simulink model "dvbs2hdlTransmitter"  (R2024b)
settings: Solver=FixedStepDiscrete  StartTime=0.0  StopTime=stopTime  RelTol=1e-3
InitFcn:
  | dvbs2hdlTxInit;
  | 
  | clear simDummyFrameNos;
StopFcn:
  | if exist('simDummyFrameNos','var')
  |    dvbs2hdlTransmitterVerify;
  | end
undefined symbols (not defined in the file or in its folder): DFLNormal, DFLShort, MODCOD, nFrames, UPL
libraries: hdlsllib x9, simulink x7, dspsrcs4 x6
CloseFcn:
  | clear curFrameBits curnPkts DFL FECFrame frameBits ...
  |     frameEndIn frameNo frameStartIn MODCOD nFrames ...
  |     pktBitsIn pktEndIn pktsSent pktStartIn pktValidIn ...
  |     PLFL Rsym stopTime StreamFormat syncWord TSorGS ...
  |     UPL
  | clear err FECFrameStr ii matframeLen matTxWaveform ...
  |     MSERe MSEIm relativeMSE RRCgain s2Config simDummyFrameNos ...
  |     simDummyFrameNums simTxWaveform tout logsout ...
  |     txObj bitsPerFrame
  | close(figure(1));
  | clear bitsIn DFLNormal DFLShort
settings Model: DataTypeOverride=Off  SimulationMode=accelerator  Creator=The MathWorks, Inc.  LastModifiedBy=daniel
settings SolverCC: AutoInsertRateTranBlk=on  MaxZcPerStep=1
settings DataIOCC: ReturnWorkspaceOutputs=off
settings OptimizationCC: BlockReduction=off  ConditionallyExecuteInputs=off  DefaultParameterBehavior=Inlined  InheritOutputTypeSmallerThanSingle=on  ReuseModelBlockBuffer=off
settings DebuggingCC: AlgebraicLoopMsg=error  SingleTaskRateTransMsg=error  SubsystemReferenceDiagnosticForUnitTest=warning
settings HardwareCC: ProdBitPerPointer=32  ProdBitPerSizeT=32  ProdBitPerPtrDiffT=32  ProdLargestAtomicFloat=None  ProdIntDivRoundTo=Undefined  ProdEndianess=Unspecified  ProdWordSize=32  ProdHWDeviceType=ASIC/FPGA->ASIC/FPGA  TargetBitPerLong=64  TargetBitPerPointer=64  TargetBitPerSizeT=64  TargetBitPerPtrDiffT=64  TargetLongLongMode=on  TargetIntDivRoundTo=Zero  TargetEndianess=LittleEndian  TargetWordSize=64  TargetHWDeviceType=Custom Processor->MATLAB Host Computer  ProdEqTarget=off
settings ModelReferenceCC: EnableRefExpFcnMdlSchedulingChecks=on
settings RTWCC: GPUComputeCapability=3.5  DLArmComputeVersion=19.05

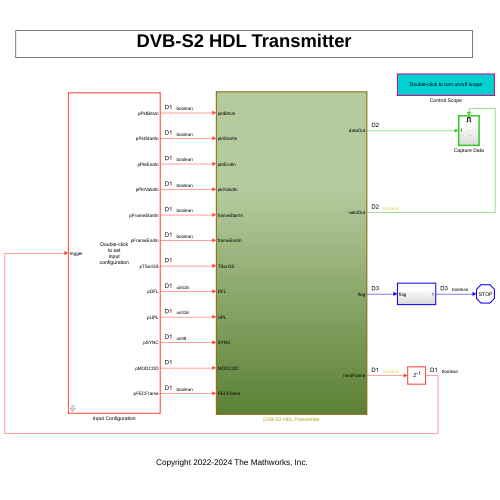
[thumbnail: Simulink's stored preview of the top-level diagram]
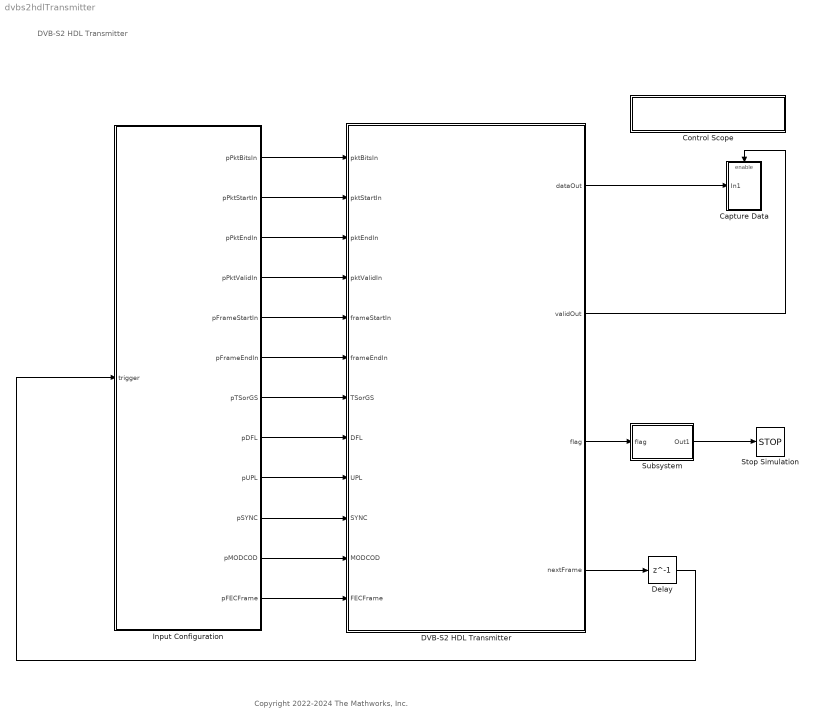
== system dvbs2hdlTransmitter ==
  note: Copyright 2022-2024 The Mathworks, Inc.
  note: DVB-S2 HDL Transmitter
  Capture Data : Subsystem
  Control Scope : Subsystem
      settings: OpenFcn=|
      | h = get_param([gcs '/Capture Data/Spectrum Analyzer'],'ScopeConfiguration');
      | 
      | h.Visible = ~h.Visible;
      | 
      | clear h;
      mask Display: disp('Double-click to turn on/off scope');
  DVB-S2 HDL Transmitter : Subsystem
  Delay : Delay  DelayLength=1
  Input Configuration : Subsystem  mask{Rsym=125e3, MODCODval=[11,17,23,28], FECFrameval=zeros(1,4), InputStreamFormat=GS, UPLval=1504}
      mask prompts: Rsym "Symbol rate:"; MODCODval "MODCOD:"; FECFrameval "FECFrame:"; InputStreamFormat "Input stream format:"; UPLval "UPL:"
      mask TypeOptions InputStreamFormat: TS | GS
      mask DialogControl DescTextVar Prompt: When Input stream format is set to TS, the UPL value is taken as 1504. The value that is set here is ignored.
      mask Display: disp(['Double-click' newline 'to set' newline 'input' newline 'configuration']);
  Stop Simulation : Stop
  Subsystem : Subsystem
      settings: LibrarySourceBlock=|
      | hdlsllib/Ports &
      | Subsystems/Subsystem
  wires:
  Input Configuration/1(pPktBitsIn) -> DVB-S2 HDL Transmitter/1(pktBitsIn)
  Input Configuration/2(pPktStartIn) -> DVB-S2 HDL Transmitter/2(pktStartIn)
  Input Configuration/3(pPktEndIn) -> DVB-S2 HDL Transmitter/3(pktEndIn)
  Input Configuration/4(pPktValidIn) -> DVB-S2 HDL Transmitter/4(pktValidIn)
  Input Configuration/5(pFrameStartIn) -> DVB-S2 HDL Transmitter/5(frameStartIn)
  Input Configuration/6(pFrameEndIn) -> DVB-S2 HDL Transmitter/6(frameEndIn)
  Input Configuration/7(pTSorGS) -> DVB-S2 HDL Transmitter/7(TSorGS)
  Input Configuration/8(pDFL) -> DVB-S2 HDL Transmitter/8(DFL)
  Input Configuration/9(pUPL) -> DVB-S2 HDL Transmitter/9(UPL)
  Input Configuration/10(pSYNC) -> DVB-S2 HDL Transmitter/10(SYNC)
  Input Configuration/11(pMODCOD) -> DVB-S2 HDL Transmitter/11(MODCOD)
  DVB-S2 HDL Transmitter/1(dataOut) -> Capture Data/1(In1)
  DVB-S2 HDL Transmitter/2(validOut) -> Capture Data/Enable
  DVB-S2 HDL Transmitter/4(nextFrame) -> Delay/1
  Input Configuration/12(pFECFrame) -> DVB-S2 HDL Transmitter/12(FECFrame)
  Delay/1 -> Input Configuration/1(trigger)
  DVB-S2 HDL Transmitter/3(flag) -> Subsystem/1(flag)
  Subsystem/1(Out1) -> Stop Simulation/1

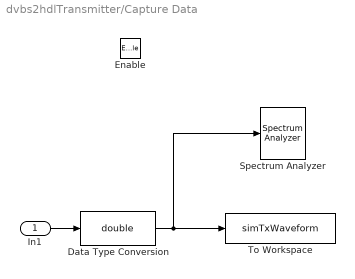
== system dvbs2hdlTransmitter/Capture Data ==
  In1 : Inport
  Enable : EnablePort
  Data Type Conversion : DataTypeConversion  OutDataTypeStr=double  SaturateOnIntegerOverflow=off  RndMeth=Floor
  Spectrum Analyzer : SpectrumAnalyzer  WindowPosition=[267.000000,736.000000,800.000000,450.000000,]  ScopeFrameLocation=window  Span=25000000  StartFrequency=-12500000  StopFrequency=12500000  AveragingMethod=Exponential  YLimits=[-78.80944125,11.88041305]  AllowFFTLengthLessThanSamplesPerUpdate=on
  To Workspace : ToWorkspace  VariableName=simTxWaveform  SampleTime=-1
      settings: Save2DSignal=2-D array (concatenate along first dimension)
  wires:
  In1/1 -> Data Type Conversion/1
  Data Type Conversion/1 -> Spectrum Analyzer/1, To Workspace/1

== system dvbs2hdlTransmitter/Control Scope ==

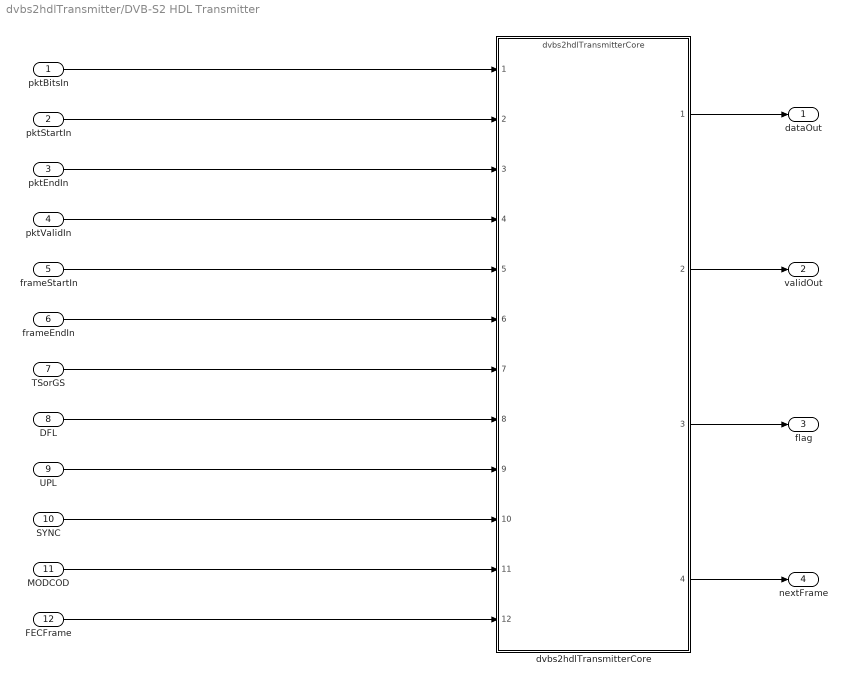
== system dvbs2hdlTransmitter/DVB-S2 HDL Transmitter ==
  pktBitsIn : Inport
  pktStartIn : Inport  Port=2
  pktEndIn : Inport  Port=3
  pktValidIn : Inport  Port=4
  frameStartIn : Inport  Port=5
  frameEndIn : Inport  Port=6
  TSorGS : Inport  Port=7
  DFL : Inport  Port=8
  UPL : Inport  Port=9
  SYNC : Inport  Port=10
  MODCOD : Inport  Port=11
  FECFrame : Inport  Port=12
  dvbs2hdlTransmitterCore : ModelReference  ModelNameDialog=dvbs2hdlTransmitterCore.slx  ModelReferenceVersion=6.8
  dataOut : Outport
  validOut : Outport  Port=2
  flag : Outport  Port=3
  nextFrame : Outport  Port=4
  wires:
  pktBitsIn/1 -> dvbs2hdlTransmitterCore/1
  pktStartIn/1 -> dvbs2hdlTransmitterCore/2
  pktEndIn/1 -> dvbs2hdlTransmitterCore/3
  pktValidIn/1 -> dvbs2hdlTransmitterCore/4
  frameStartIn/1 -> dvbs2hdlTransmitterCore/5
  frameEndIn/1 -> dvbs2hdlTransmitterCore/6
  TSorGS/1 -> dvbs2hdlTransmitterCore/7
  DFL/1 -> dvbs2hdlTransmitterCore/8
  UPL/1 -> dvbs2hdlTransmitterCore/9
  SYNC/1 -> dvbs2hdlTransmitterCore/10
  MODCOD/1 -> dvbs2hdlTransmitterCore/11
  FECFrame/1 -> dvbs2hdlTransmitterCore/12
  dvbs2hdlTransmitterCore/2 -> validOut/1
  dvbs2hdlTransmitterCore/1 -> dataOut/1
  dvbs2hdlTransmitterCore/4 -> nextFrame/1
  dvbs2hdlTransmitterCore/3 -> flag/1

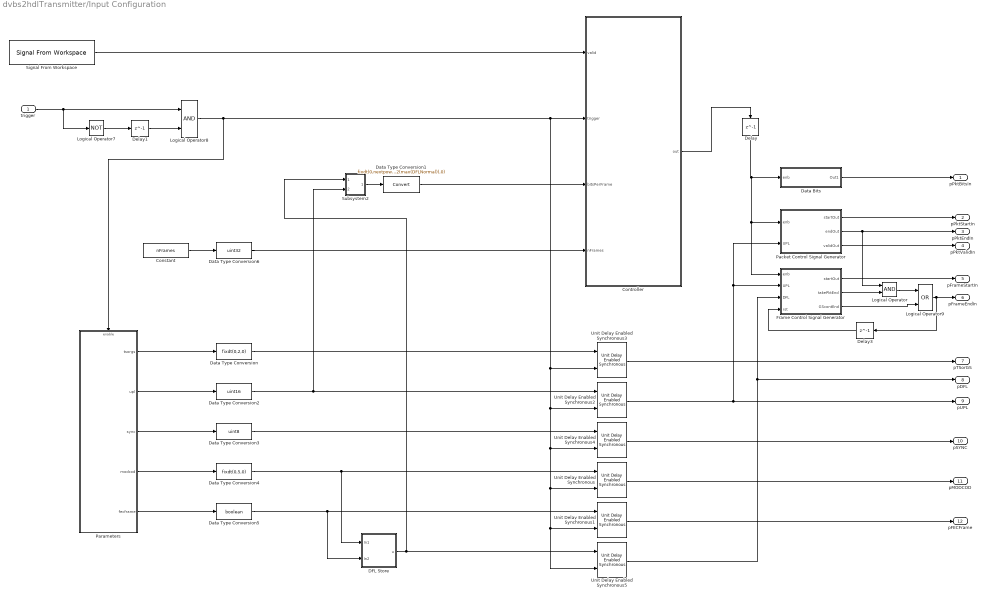
== system dvbs2hdlTransmitter/Input Configuration ==
  trigger : Inport
  Constant : Constant  Value=nFrames  SampleTime=-1
  Controller : MATLAB Function  TreatAsAtomicUnit=on
  DFL Store : Subsystem
  Data Bits : Subsystem
  Data Type Conversion : DataTypeConversion  OutDataTypeStr=fixdt(0,2,0)  SaturateOnIntegerOverflow=off  RndMeth=Floor
  Data Type Conversion1 : DataTypeConversion  OutDataTypeStr=fixdt(0,nextpow2(max(DFLNormal)),0)  SaturateOnIntegerOverflow=off  RndMeth=Floor
  Data Type Conversion2 : DataTypeConversion  OutDataTypeStr=uint16  SaturateOnIntegerOverflow=off  RndMeth=Floor
  Data Type Conversion3 : DataTypeConversion  OutDataTypeStr=uint8  SaturateOnIntegerOverflow=off  RndMeth=Floor
  Data Type Conversion4 : DataTypeConversion  OutDataTypeStr=fixdt(0,5,0)  SaturateOnIntegerOverflow=off  RndMeth=Floor
  Data Type Conversion5 : DataTypeConversion  OutDataTypeStr=boolean  SaturateOnIntegerOverflow=off  RndMeth=Floor
  Data Type Conversion6 : DataTypeConversion  OutDataTypeStr=uint32  SaturateOnIntegerOverflow=off  RndMeth=Floor
  Delay : Delay  DelayLength=1
  Delay1 : Delay  DelayLength=1
  Delay3 : Delay  DelayLength=1
  Frame Control Signal Generator : Subsystem
  Logical Operator : Logic  AllPortsSameDT=off  OutDataTypeStr=boolean
  Logical Operator7 : Logic  Operator=NOT  AllPortsSameDT=off  OutDataTypeStr=boolean
  Logical Operator8 : Logic  AllPortsSameDT=off  OutDataTypeStr=boolean
  Logical Operator9 : Logic  Operator=OR  AllPortsSameDT=off  OutDataTypeStr=boolean
  Packet Control Signal Generator : Subsystem
  Parameters : Subsystem
  Signal From Workspace : dspsrcs4/Signal From Workspace  X=true  Ts=1/(Rsym*8)  nsamps=1  OutputAfterFinalValue=Cyclic repetition  ignoreOrWarnInputAndFrameLengths=off  OutputFrames=off
  Subsystem2 : Subsystem
  Unit Delay Enabled Synchronous{,1..5} (6 alike) : hdlsllib/Discrete/Unit Delay Enabled Synchronous  InitialCondition=0.0  SampleTime=-1
  pPktBitsIn : Outport
  pPktStartIn : Outport  Port=2
  pPktEndIn : Outport  Port=3
  pPktValidIn : Outport  Port=4
  pFrameStartIn : Outport  Port=5
  pFrameEndIn : Outport  Port=6
  pTSorGS : Outport  Port=7
  pDFL : Outport  Port=8
  pUPL : Outport  Port=9
  pSYNC : Outport  Port=10
  pMODCOD : Outport  Port=11
  pFECFrame : Outport  Port=12
  wires:
  Controller/1(out) -> Delay/1
  Data Type Conversion4/1 -> DFL Store/1(In1), Unit Delay Enabled Synchronous/1
  Data Type Conversion5/1 -> Unit Delay Enabled Synchronous1/1, DFL Store/2(In2)
  Data Type Conversion2/1 -> Unit Delay Enabled Synchronous2/1, Subsystem2/2(UPL)
  Signal From Workspace/1 -> Controller/1(valid)
  Unit Delay Enabled Synchronous2/1 -> pUPL/1, Packet Control Signal Generator/2(UPL), Frame Control Signal Generator/2(UPL)
  Frame Control Signal Generator/2(takePktEnd) -> Logical Operator/2
  Packet Control Signal Generator/2(endOut) -> pPktEndIn/1, Logical Operator/1
  Data Type Conversion/1 -> Unit Delay Enabled Synchronous3/1
  Logical Operator8/1 -> Parameters/Enable, Unit Delay Enabled Synchronous3/2, Unit Delay Enabled Synchronous1/2, Unit Delay Enabled Synchronous5/2, Unit Delay Enabled Synchronous/2, Unit Delay Enabled Synchronous4/2, Unit Delay Enabled Synchronous2/2, Controller/2(trigger)
  Data Bits/1(Out1) -> pPktBitsIn/1
  Packet Control Signal Generator/1(startOut) -> pPktStartIn/1
  Packet Control Signal Generator/3(validOut) -> pPktValidIn/1
  Frame Control Signal Generator/1(startOut) -> pFrameStartIn/1
  Logical Operator9/1 -> pFrameEndIn/1, Delay3/1
  Data Type Conversion3/1 -> Unit Delay Enabled Synchronous4/1
  Parameters/2(upl) -> Data Type Conversion2/1
  Parameters/4(modcod) -> Data Type Conversion4/1
  Parameters/5(fecframe) -> Data Type Conversion5/1
  Parameters/1(tsorgs) -> Data Type Conversion/1
  Parameters/3(sync) -> Data Type Conversion3/1
  DFL Store/1(u) -> Subsystem2/1(DFL), Unit Delay Enabled Synchronous5/1
  Unit Delay Enabled Synchronous5/1 -> pDFL/1, Frame Control Signal Generator/3(DFL)
  Unit Delay Enabled Synchronous3/1 -> pTSorGS/1
  Unit Delay Enabled Synchronous/1 -> pMODCOD/1
  Unit Delay Enabled Synchronous4/1 -> pSYNC/1
  Unit Delay Enabled Synchronous1/1 -> pFECFrame/1
  Delay/1 -> Frame Control Signal Generator/1(enb), Packet Control Signal Generator/1(enb), Data Bits/1(enb)
  trigger/1 -> Logical Operator7/1, Logical Operator8/1
  Delay1/1 -> Logical Operator8/2
  Logical Operator7/1 -> Delay1/1
  Delay3/1 -> Frame Control Signal Generator/4(rst)
  Logical Operator/1 -> Logical Operator9/1
  Frame Control Signal Generator/3(GScontEnd) -> Logical Operator9/2
  Constant/1 -> Data Type Conversion6/1
  Data Type Conversion1/1 -> Controller/3(bitsPerFrame)
  Subsystem2/1(Out1) -> Data Type Conversion1/1
  Data Type Conversion6/1 -> Controller/4(nFrames)

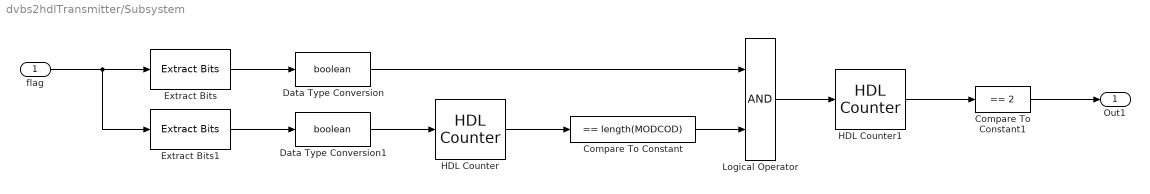
== system dvbs2hdlTransmitter/Subsystem ==
  flag : Inport
  Compare To Constant : simulink/Logic and Bit Operations/Compare To Constant  relop===  const=length(MODCOD)  OutDataTypeStr=boolean
  Compare To Constant1 : simulink/Logic and Bit Operations/Compare To Constant  relop===  const=2  OutDataTypeStr=boolean
  Data Type Conversion : DataTypeConversion  OutDataTypeStr=boolean  SaturateOnIntegerOverflow=off  RndMeth=Floor
  Data Type Conversion1 : DataTypeConversion  OutDataTypeStr=boolean  SaturateOnIntegerOverflow=off  RndMeth=Floor
  Extract Bits : simulink/Logic and Bit Operations/Extract Bits  bitsToExtract=Upper half  numBits=8  bitIdxRange=[0 7]  outScalingMode=Treat bit field as an integer
  Extract Bits1 : simulink/Logic and Bit Operations/Extract Bits  bitsToExtract=Lower half  numBits=8  bitIdxRange=[0 7]  outScalingMode=Treat bit field as an integer
  HDL Counter : hdlsllib/Sources/HDL Counter  CountType=Free running  CountInit=0  CountStep=1  CountMax=25  CountFromType=Initial value  CountFrom=0  CountResetPort=off  CountLoadPort=off  CountEnbPort=on  CountDirPort=off  CountHitOutputPort=off  CountDataType=Unsigned  CountWordLen=32  CountFracLen=0  CountSampTime=1
  HDL Counter1 : hdlsllib/Sources/HDL Counter  CountType=Free running  CountInit=0  CountStep=1  CountMax=25  CountFromType=Initial value  CountFrom=0  CountResetPort=off  CountLoadPort=off  CountEnbPort=on  CountDirPort=off  CountHitOutputPort=off  CountDataType=Unsigned  CountWordLen=32  CountFracLen=0  CountSampTime=1
  Logical Operator : Logic  AllPortsSameDT=off  OutDataTypeStr=boolean
  Out1 : Outport  VectorParamsAs1DForOutWhenUnconnected=off
  wires:
  flag/1 -> Extract Bits1/1, Extract Bits/1
  Extract Bits/1 -> Data Type Conversion/1
  Extract Bits1/1 -> Data Type Conversion1/1
  Data Type Conversion1/1 -> HDL Counter/1
  HDL Counter/1 -> Compare To Constant/1
  Data Type Conversion/1 -> Logical Operator/1
  Compare To Constant/1 -> Logical Operator/2
  Logical Operator/1 -> HDL Counter1/1
  HDL Counter1/1 -> Compare To Constant1/1
  Compare To Constant1/1 -> Out1/1

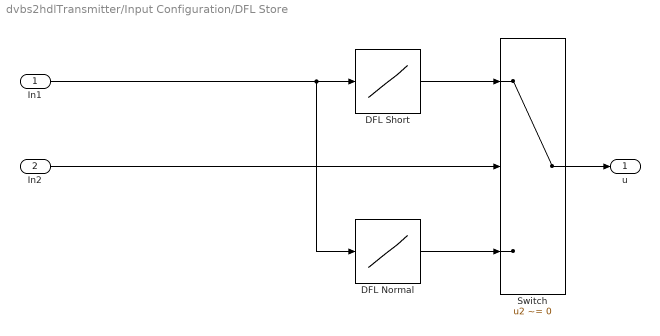
== system dvbs2hdlTransmitter/Input Configuration/DFL Store ==
  In1 : Inport
  In2 : Inport  Port=2
  DFL Normal : Lookup_n-D  NumberOfTableDimensions=1  LookupTableObject=''  BreakpointsForDimension1=0:28  BreakpointsForDimension1FirstPoint=10  BreakpointsForDimension2FirstPoint=10  BreakpointsForDimension1Spacing=12  BreakpointsForDimension2Spacing=12  IndexSearchMethod=Evenly spaced points  Table=[0 DFLNormal]  TableDataTypeStr=fixdt(0,nextpow2(max(DFLNormal)),0)  InterpMethod=Flat  DiagnosticForOutOfRangeInput=Error  InternalRulePriority=Speed  OutDataTypeStr=fixdt(0,nextpow2(max(DFLNormal)),0)  RndMeth=Simplest
  DFL Short : Lookup_n-D  NumberOfTableDimensions=1  LookupTableObject=''  BreakpointsForDimension1=0:28  BreakpointsForDimension1FirstPoint=10  BreakpointsForDimension2FirstPoint=10  BreakpointsForDimension1Spacing=12  BreakpointsForDimension2Spacing=12  IndexSearchMethod=Evenly spaced points  Table=[0 DFLShort]  TableDataTypeStr=fixdt(0,nextpow2(max(DFLNormal)),0)  InterpMethod=Flat  DiagnosticForOutOfRangeInput=Error  InternalRulePriority=Speed  OutDataTypeStr=fixdt(0,nextpow2(max(DFLNormal)),0)  RndMeth=Simplest
  Switch : Switch  Criteria=u2 ~= 0  SaturateOnIntegerOverflow=off  InputSameDT=off
  u : Outport
  wires:
  DFL Normal/1 -> Switch/3
  In2/1 -> Switch/2
  Switch/1 -> u/1
  DFL Short/1 -> Switch/1
  In1/1 -> DFL Normal/1, DFL Short/1

== system dvbs2hdlTransmitter/Input Configuration/Data Bits ==
  enb : Inport
  Constant1 : Constant  Value=0  OutDataTypeStr=Inherit: Inherit via back propagation  SampleTime=-1
  Subsystem : Subsystem
  Switch1 : Switch  Criteria=u2 > Threshold  SaturateOnIntegerOverflow=off  InputSameDT=off
  Out1 : Outport
  wires:
  enb/1 -> Switch1/2, Subsystem/Enable
  Constant1/1 -> Switch1/3
  Subsystem/1(Outport) -> Switch1/1
  Switch1/1 -> Out1/1

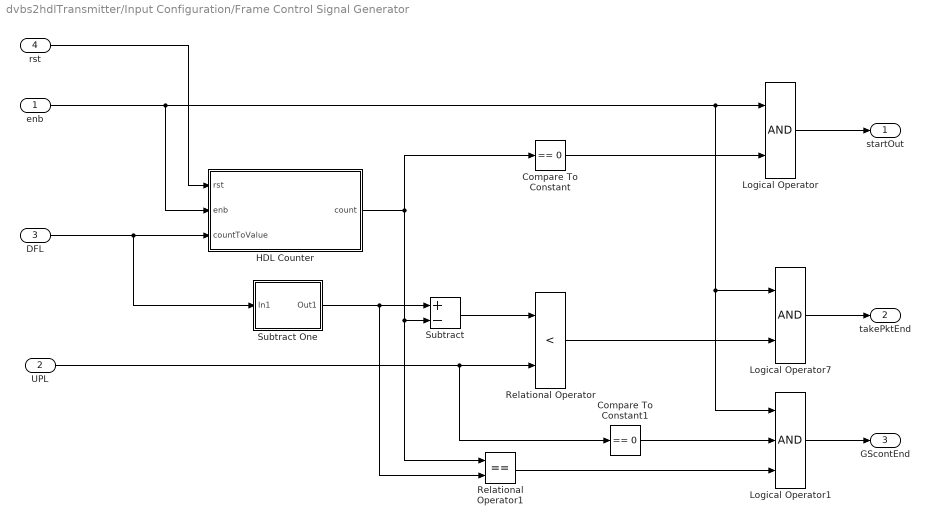
== system dvbs2hdlTransmitter/Input Configuration/Frame Control Signal Generator ==
  enb : Inport
  UPL : Inport  Port=2
  DFL : Inport  Port=3
  rst : Inport  Port=4
  Compare To Constant : simulink/Logic and Bit Operations/Compare To Constant  relop===  const=0  OutDataTypeStr=boolean
  Compare To Constant1 : simulink/Logic and Bit Operations/Compare To Constant  relop===  const=0  OutDataTypeStr=boolean
  HDL Counter : MATLAB Function  TreatAsAtomicUnit=on
  Logical Operator : Logic  AllPortsSameDT=off  OutDataTypeStr=boolean
  Logical Operator1 : Logic  Inputs=3  AllPortsSameDT=off  OutDataTypeStr=boolean
  Logical Operator7 : Logic  AllPortsSameDT=off  OutDataTypeStr=boolean
  Relational Operator : RelationalOperator  Operator=<  OutDataTypeStr=boolean  RndMeth=Simplest  InputSameDT=off
  Relational Operator1 : RelationalOperator  Operator===  OutDataTypeStr=boolean  RndMeth=Simplest  InputSameDT=off
  Subtract : Sum  Inputs=+-  OutDataTypeStr=Inherit: Same as first input
  Subtract One : Subsystem
  startOut : Outport  VectorParamsAs1DForOutWhenUnconnected=off
  takePktEnd : Outport  Port=2  VectorParamsAs1DForOutWhenUnconnected=off
  GScontEnd : Outport  Port=3  VectorParamsAs1DForOutWhenUnconnected=off
  wires:
  Subtract One/1(Out1) -> Relational Operator1/2, Subtract/1
  enb/1 -> Logical Operator/1, Logical Operator1/1, Logical Operator7/1, HDL Counter/2(enb)
  Compare To Constant/1 -> Logical Operator/2
  Logical Operator/1 -> startOut/1
  Logical Operator7/1 -> takePktEnd/1
  HDL Counter/1(count) -> Relational Operator1/1, Subtract/2, Compare To Constant/1
  Subtract/1 -> Relational Operator/1
  rst/1 -> HDL Counter/1(rst)
  UPL/1 -> Compare To Constant1/1, Relational Operator/2
  DFL/1 -> Subtract One/1(In1), HDL Counter/3(countToValue)
  Relational Operator1/1 -> Logical Operator1/3
  Relational Operator/1 -> Logical Operator7/2
  Logical Operator1/1 -> GScontEnd/1
  Compare To Constant1/1 -> Logical Operator1/2

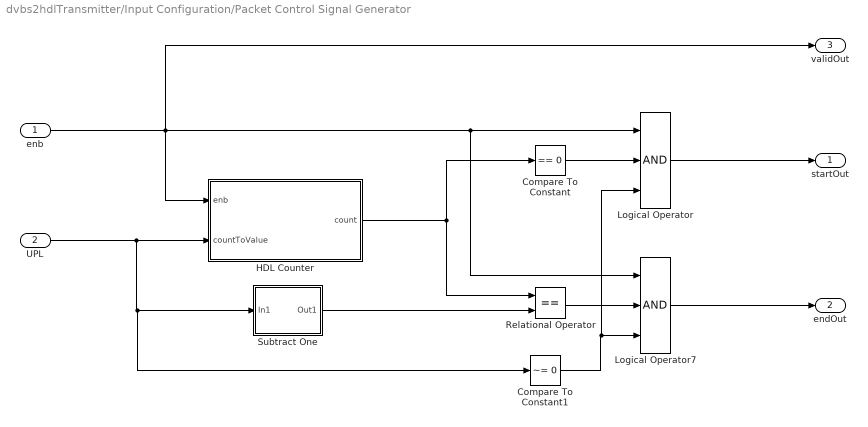
== system dvbs2hdlTransmitter/Input Configuration/Packet Control Signal Generator ==
  enb : Inport
  UPL : Inport  Port=2
  Compare To Constant : simulink/Logic and Bit Operations/Compare To Constant  relop===  const=0  OutDataTypeStr=boolean
  Compare To Constant1 : hdlsllib/Logic and Bit Operations/Compare To Constant  relop=~=  const=0  OutDataTypeStr=boolean
  HDL Counter : MATLAB Function  TreatAsAtomicUnit=on
  Logical Operator : Logic  Inputs=3  AllPortsSameDT=off  OutDataTypeStr=boolean
  Logical Operator7 : Logic  Inputs=3  AllPortsSameDT=off  OutDataTypeStr=boolean
  Relational Operator : RelationalOperator  Operator===  OutDataTypeStr=boolean  RndMeth=Simplest  InputSameDT=off
  Subtract One : Subsystem
  startOut : Outport  VectorParamsAs1DForOutWhenUnconnected=off
  endOut : Outport  Port=2  VectorParamsAs1DForOutWhenUnconnected=off
  validOut : Outport  Port=3  VectorParamsAs1DForOutWhenUnconnected=off
  wires:
  HDL Counter/1(count) -> Relational Operator/1, Compare To Constant/1
  Logical Operator7/1 -> endOut/1
  Logical Operator/1 -> startOut/1
  Compare To Constant/1 -> Logical Operator/2
  enb/1 -> validOut/1, HDL Counter/1(enb), Logical Operator7/1, Logical Operator/1
  UPL/1 -> Subtract One/1(In1), Compare To Constant1/1, HDL Counter/2(countToValue)
  Relational Operator/1 -> Logical Operator7/2
  Subtract One/1(Out1) -> Relational Operator/2
  Compare To Constant1/1 -> Logical Operator/3, Logical Operator7/3

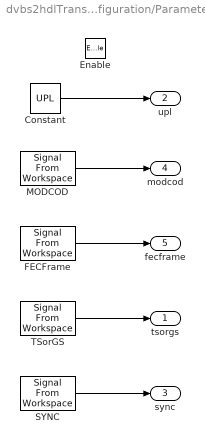
== system dvbs2hdlTransmitter/Input Configuration/Parameters ==
  Enable : EnablePort
  Constant : Constant  Value=UPL  SampleTime=-1
  FECFrame : dspsrcs4/Signal From Workspace  X=FECFrame  Ts=1/(Rsym*8)  nsamps=1  OutputAfterFinalValue=Setting to zero  ignoreOrWarnInputAndFrameLengths=off  OutputFrames=off
  MODCOD : dspsrcs4/Signal From Workspace  X=MODCOD  Ts=1/(Rsym*8)  nsamps=1  OutputAfterFinalValue=Holding final value  ignoreOrWarnInputAndFrameLengths=off  OutputFrames=off
  SYNC : dspsrcs4/Signal From Workspace  X=syncWord  Ts=1/(Rsym*8)  nsamps=1  OutputAfterFinalValue=Holding final value  ignoreOrWarnInputAndFrameLengths=off  OutputFrames=off
  TSorGS : dspsrcs4/Signal From Workspace  X=TSorGS  Ts=1/(Rsym*8)  nsamps=1  OutputAfterFinalValue=Holding final value  ignoreOrWarnInputAndFrameLengths=off  OutputFrames=off
  tsorgs : Outport
  upl : Outport  Port=2
  sync : Outport  Port=3
  modcod : Outport  Port=4
  fecframe : Outport  Port=5
  wires:
  TSorGS/1 -> tsorgs/1
  FECFrame/1 -> fecframe/1
  Constant/1 -> upl/1
  SYNC/1 -> sync/1
  MODCOD/1 -> modcod/1

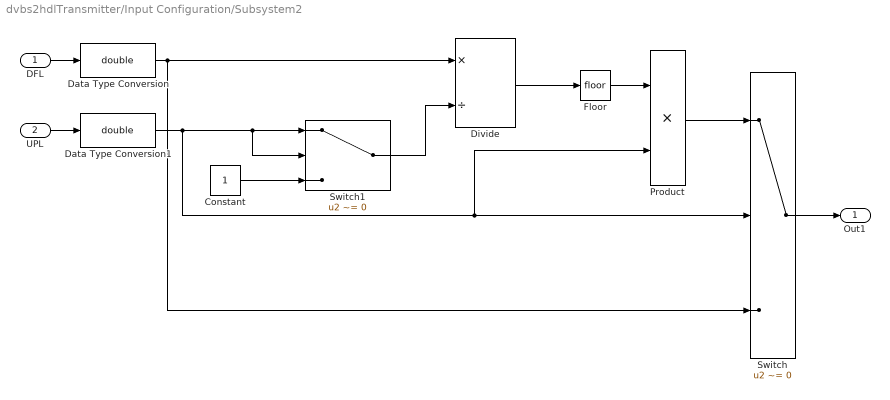
== system dvbs2hdlTransmitter/Input Configuration/Subsystem2 ==
  DFL : Inport
  UPL : Inport  Port=2
  Constant : Constant  OutDataTypeStr=Inherit: Inherit via back propagation  SampleTime=-1
  Data Type Conversion : DataTypeConversion  OutDataTypeStr=double  SaturateOnIntegerOverflow=off  RndMeth=Floor
  Data Type Conversion1 : DataTypeConversion  OutDataTypeStr=double  SaturateOnIntegerOverflow=off  RndMeth=Floor
  Divide : Product  Inputs=*/
  Floor : Rounding
  Product : Product
  Switch : Switch  Criteria=u2 ~= 0  SaturateOnIntegerOverflow=off  InputSameDT=off
  Switch1 : Switch  Criteria=u2 ~= 0  SaturateOnIntegerOverflow=off  InputSameDT=off
  Out1 : Outport
  wires:
  Floor/1 -> Product/1
  Product/1 -> Switch/1
  DFL/1 -> Data Type Conversion/1
  UPL/1 -> Data Type Conversion1/1
  Switch/1 -> Out1/1
  Divide/1 -> Floor/1
  Data Type Conversion1/1 -> Switch1/2, Switch1/1, Product/2, Switch/2
  Constant/1 -> Switch1/3
  Data Type Conversion/1 -> Switch/3, Divide/1
  Switch1/1 -> Divide/2

== system dvbs2hdlTransmitter/Input Configuration/Data Bits/Subsystem ==
  Enable : EnablePort
  Signal From Workspace1 : dspsrcs4/Signal From Workspace  X=bitsIn  Ts=1/(Rsym*8)  nsamps=1  OutputAfterFinalValue=Setting to zero  ignoreOrWarnInputAndFrameLengths=off  OutputFrames=off
  Outport : Outport
  wires:
  Signal From Workspace1/1 -> Outport/1

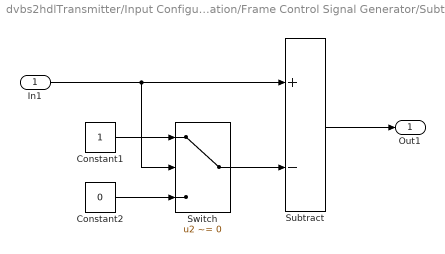
== system dvbs2hdlTransmitter/Input Configuration/Frame Control Signal Generator/Subtract One ==
  In1 : Inport
  Constant1 : Constant  OutDataTypeStr=fixdt(0,1,0)  SampleTime=-1
  Constant2 : Constant  Value=0  OutDataTypeStr=fixdt(0,1,0)  SampleTime=-1
  Subtract : Sum  Inputs=+-  OutDataTypeStr=Inherit: Same as first input
  Switch : Switch  Criteria=u2 ~= 0  SaturateOnIntegerOverflow=off  InputSameDT=off
  Out1 : Outport
  wires:
  In1/1 -> Switch/2, Subtract/1
  Switch/1 -> Subtract/2
  Constant1/1 -> Switch/1
  Constant2/1 -> Switch/3
  Subtract/1 -> Out1/1

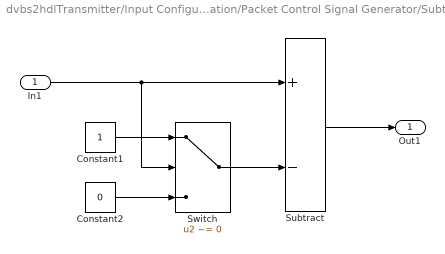
== system dvbs2hdlTransmitter/Input Configuration/Packet Control Signal Generator/Subtract One ==
  In1 : Inport
  Constant1 : Constant  OutDataTypeStr=fixdt(0,1,0)  SampleTime=-1
  Constant2 : Constant  Value=0  OutDataTypeStr=fixdt(0,1,0)  SampleTime=-1
  Subtract : Sum  Inputs=+-  OutDataTypeStr=Inherit: Same as first input
  Switch : Switch  Criteria=u2 ~= 0  SaturateOnIntegerOverflow=off  InputSameDT=off
  Out1 : Outport
  wires:
  In1/1 -> Switch/2, Subtract/1
  Switch/1 -> Subtract/2
  Constant1/1 -> Switch/1
  Constant2/1 -> Switch/3
  Subtract/1 -> Out1/1

== matlab function dvbs2hdlTransmitter/Input Configuration/Packet Control Signal Generator/HDL Counter ==
  data: enb input; count output; countToValue input
function count = fcn(enb,countToValue)
%#codegen

  persistent countState;
  if isempty(countState)
      countState = cast(0,'like',countToValue);
  end

  count = countState;

  if enb && (countToValue ~= 0)
      if countState == countToValue - 1
          countState(:) = 0;
      else
          countState(:) = countState + 1;
      end
  end

end

== matlab function dvbs2hdlTransmitter/Input Configuration/Frame Control Signal Generator/HDL Counter ==
  data: rst input; enb input; count output; countToValue input
function count = fcn(rst,enb,countToValue)
%#codegen

  persistent countState;
  if isempty(countState)
      countState = cast(0,'like',countToValue);
  end
  
  count = countState;

  if enb && (countToValue ~= 0)
      if countState == countToValue - 1
          countState(:) = 0;
      else
          countState(:) = countState + 1;
      end
  end

  if rst
      countState(:) = 0;
  end

end

== matlab function dvbs2hdlTransmitter/Input Configuration/Controller ==
  data: valid input; trigger input; bitsPerFrame input; nFrames input; out output
function out = fcn(valid,trigger,bitsPerFrame,nFrames)
%#codegen

    persistent frameNo count countActive ;
    if isempty(count)
        count = cast(0,'like',bitsPerFrame);
        frameNo = 0;
        countActive = false;
    end

    if trigger 
        frameNo(:) = frameNo + 1;
        countActive = true;
    end

    if valid
        if (frameNo <= nFrames)
            if countActive
                if count == bitsPerFrame
                    countActive = false;
                    count(:) = 0;
                    out = false;
                else
                    count(:) = count + 1;
                    out = true;
                end
            else
                out = false;
            end
        else
            out = false;
        end
    else
        out = false;
    end
    
end
